simulink model "EstimatingFunctionForLine"  (R2019b)
settings: Solver=FixedStepAuto  StartTime=0.0  StopTime=6  RelTol=1e-3  EnableMultiTasking=on
libraries: legoev3lib x4
settings Model: ExtModeTrigDuration=2  Creator=nikit  LastModifiedBy=nikit
settings SolverCC: PositivePriorityOrder=on
settings OptimizationCC: EnhancedBackFolding=on  PassReuseOutputArgsAs=Individual arguments  ZeroExternalMemoryAtStartup=off  ZeroInternalMemoryAtStartup=off  MaxStackSize=64  OptimizeBlockOrder=speed  DifferentSizesBufferReuse=on  OptimizationCustomize=off  EfficientTunableParamExpr=on
settings DebuggingCC: ParameterTunabilityLossMsg=error
settings HardwareCC: ProdBitPerPointer=32  ProdBitPerSizeT=32  ProdBitPerPtrDiffT=32  ProdLargestAtomicInteger=Long  ProdWordSize=32  ProdHWDeviceType=ARM Compatible->ARM 9
settings SFSimCC: MATLABDynamicMemAlloc=off
settings RTWCC: SystemTargetFile=ert.tlc  HardwareBoard=LEGO MINDSTORMS EV3  TLCOptions="-aInlineSetEventsForThisBaseRateFcn=TLC_FALSE -aSuppressMultiTaskScheduler=TLC_FALSE  -aRateBasedStepFcn=0"  TemplateMakefile=ert_default_tmf  GenerateReport=on  Toolchain=Sourcery G++ Lite v2009q3  IncludeHyperlinkInReport=on  LaunchReport=on  GenerateTraceInfo=on  GenerateTraceReport=on  GenerateTraceReportSl=on  GenerateTraceReportSf=on  GenerateTraceReportEml=on
settings CodeAppCC: ForceParamTrailComments=on  IgnoreCustomStorageClasses=off  OperatorAnnotations=on  SimulinkDataObjDesc=on  SFDataObjDesc=on  InsertBlockDesc=on
settings ERTTargetCC: SupportContinuousTime=on  SupportVariableSizeSignals=on

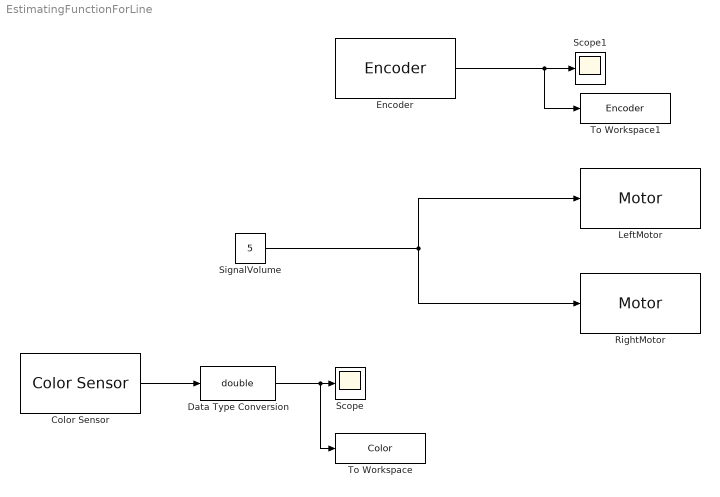
== system EstimatingFunctionForLine ==
  Color Sensor : legoev3lib/Color Sensor  portNumber=2  mode=Reflected light intensity  sampleTime=0.1
      settings: SourceProductName=Simulink Support Package for LEGO MINDSTORMS EV3 Hardware  SourceProductBaseCode=LEGOEV3
  Data Type Conversion : DataTypeConversion  OutDataTypeStr=double
  Encoder : legoev3lib/Encoder  portNumber=A  opMode=No reset  sampleTime=0.1
      settings: SourceProductName=Simulink Support Package for LEGO MINDSTORMS EV3 Hardware  SourceProductBaseCode=LEGOEV3
  LeftMotor : legoev3lib/Motor  sportNumber=A  sstopAction=Brake
  RightMotor : legoev3lib/Motor  sportNumber=D  sstopAction=Brake
  Scope : Scope
  Scope1 : Scope
  SignalVolume : Constant  Value=5
  To Workspace : ToWorkspace  VariableName=Color  SampleTime=-1
      settings: Save2DSignal=2-D array (concatenate along first dimension)
  To Workspace1 : ToWorkspace  VariableName=Encoder  SampleTime=-1
      settings: Save2DSignal=2-D array (concatenate along first dimension)
  wires:
  SignalVolume/1 -> RightMotor/1, LeftMotor/1
  Color Sensor/1 -> Data Type Conversion/1
  Encoder/1 -> To Workspace1/1, Scope1/1
  Data Type Conversion/1 -> To Workspace/1, Scope/1
